simulink model "Tuning_Circuit"  (R2020b)
settings: Solver=VariableStepAuto  StartTime=0.0  StopTime=2952  MaxStep=5/60  RelTol=0.0001
values from neighbouring files (symbols this model uses):
  K = kstat(z)    [G_Fit.m]
  tau1 = [tau1v(r) 1]    [G_Fit.m]
  tau2 = [tau2v(c) 1]    [G_Fit.m]
settings Model: Creator=andre  LastModifiedBy=andre

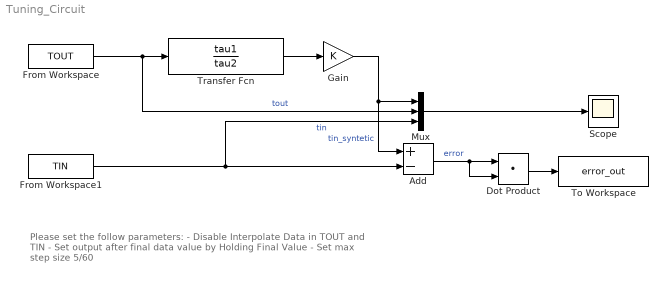
== system Tuning_Circuit ==
  note: Please set the follow parameters:
      | - Disable Interpolate Data in TOUT and TIN
      | - Set output after final data value by Holding Final Value
      | - Set max step size 5/60
  Add : Sum  Inputs=+-
  Dot Product : DotProduct  InputSameDT=on  OutDataTypeStr=Inherit: Inherit via internal rule
  From Workspace : FromWorkspace  VariableName=TOUT  Interpolate=off  ZeroCross=off  OutputAfterFinalValue=Holding final value
  From Workspace1 : FromWorkspace  VariableName=TIN  Interpolate=off  ZeroCross=off  OutputAfterFinalValue=Holding final value
  Gain : Gain  Gain=K
  Mux : Mux  Inputs=3
  Scope : Scope
  To Workspace : ToWorkspace  VariableName=error_out  SaveFormat=Timeseries  SampleTime=-1
  Transfer Fcn : TransferFcn  Numerator=tau1  Denominator=tau2
  wires:
  Mux/1 -> Scope/1
  Add/1 -> Dot Product/2, Dot Product/1  "error"
  Dot Product/1 -> To Workspace/1
  From Workspace/1 -> Mux/2, Transfer Fcn/1  "tout"
  From Workspace1/1 -> Mux/3, Add/2  "tin"
  Transfer Fcn/1 -> Gain/1
  Gain/1 -> Add/1, Mux/1  "tin_syntetic"
